simulink model "PD_teste"  (R2017b)
settings: Solver=ode45  StartTime=0.0  StopTime=5  RelTol=1e-3
settings Model: Creator=fernandopassold  LastModifiedBy=fernandopassold

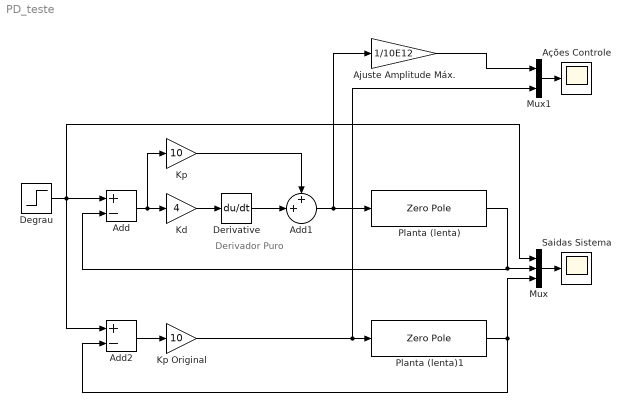
== system PD_teste ==
  note: Derivador
      | Puro
  Add : Sum  Inputs=+-
  Add1 : Sum  Inputs=++|
  Add2 : Sum  Inputs=+-
  Ajuste Amplitude Máx. : Gain  Gain=1/10E12
  Ações Controle : Scope
  Degrau : Step  SampleTime=0
  Derivative : Derivative
  Kd : Gain  Gain=4
  Kp : Gain  Gain=10
  Kp Original : Gain  Gain=10
  Mux : Mux  Inputs=3
  Mux1 : Mux  Inputs=2
  Planta (lenta) : ZeroPole  Zeros=[ ]  Poles=[-0.25]  Gain=1/4
  Planta (lenta)1 : ZeroPole  Zeros=[ ]  Poles=[-0.25]  Gain=1/4
  Saidas Sistema : Scope
  wires:
  Mux/1 -> Saidas Sistema/1
  Planta (lenta)/1 -> Add/2, Mux/2
  Add/1 -> Kp/1, Kd/1
  Kd/1 -> Derivative/1
  Add1/1 -> Ajuste Amplitude Máx./1, Planta (lenta)/1
  Derivative/1 -> Add1/2
  Kp/1 -> Add1/1
  Mux1/1 -> Ações Controle/1
  Degrau/1 -> Mux/1, Add/1, Add2/1
  Planta (lenta)1/1 -> Mux/3, Add2/2
  Add2/1 -> Kp Original/1
  Kp Original/1 -> Mux1/2, Planta (lenta)1/1
  Ajuste Amplitude Máx./1 -> Mux1/1
